simulink model "Assignment2Problem1_1"  (R2017b)
settings: Solver=VariableStepAuto  StartTime=0.0  StopTime=10.0  RelTol=1e-3
values from neighbouring files (symbols this model uses):
  A = [-4 5; 0 1]    [Assignment2Problem1.m]
  B = [0; 1]    [Assignment2Problem1.m]
  C = [1 1]    [Assignment2Problem1.m]
  D = 2    [Assignment2Problem1.m]
  x0 = [1; 2]    [Assignment2Problem1.m]
settings Model: Creator=alexbenasutti  LastModifiedBy=alexbenasutti

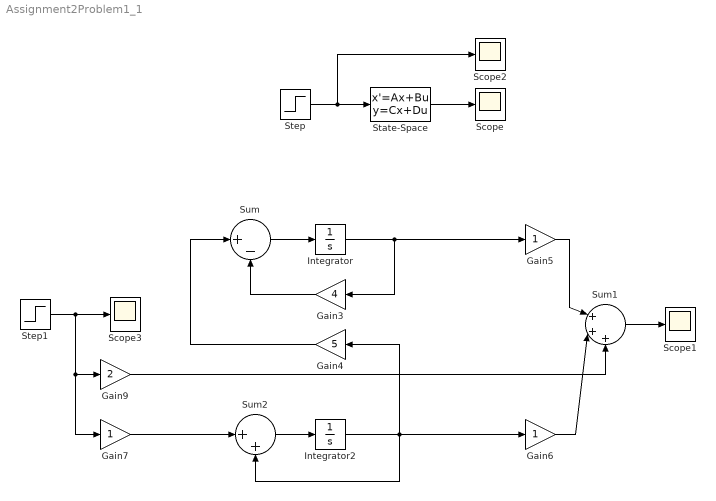
== system Assignment2Problem1_1 ==
  Gain3 : Gain  Gain=4
  Gain4 : Gain  Gain=5
  Gain5 : Gain
  Gain6 : Gain
  Gain7 : Gain
  Gain9 : Gain  Gain=2
  Integrator : Integrator  InitialCondition=1
  Integrator2 : Integrator  InitialCondition=2
  Scope{,1..3} (4 alike) : Scope
  State-Space : StateSpace  A=A  B=B  C=C  D=D  InitialCondition=x0
  Step : Step  SampleTime=0
  Step1 : Step  SampleTime=0
  Sum : Sum  Inputs=|+-
  Sum1 : Sum  Inputs=|+++
  Sum2 : Sum  Inputs=|++
  wires:
  Step/1 -> Scope2/1, State-Space/1
  State-Space/1 -> Scope/1
  Sum/1 -> Integrator/1
  Sum1/1 -> Scope1/1
  Gain6/1 -> Sum1/2
  Gain5/1 -> Sum1/1
  Step1/1 -> Scope3/1, Gain9/1, Gain7/1
  Sum2/1 -> Integrator2/1
  Gain7/1 -> Sum2/1
  Integrator2/1 -> Gain4/1, Gain6/1, Sum2/2
  Gain9/1 -> Sum1/3
  Integrator/1 -> Gain3/1, Gain5/1
  Gain3/1 -> Sum/2
  Gain4/1 -> Sum/1
